simulink model "untitled"  (Simulink 7.5)
settings: Solver=ode45  StartTime=0.0  StopTime=100.0  RelTol=1e-3
settings Model: Creator=psoltysiak  LastModifiedBy=Soltys
settings DebuggingCC: StrictBusMsg=Warning

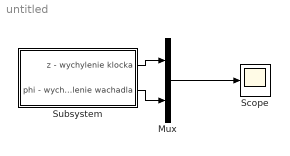
== system untitled ==
  Mux : Mux  Inputs=2
  Scope : Scope
  Subsystem : Subsystem  mask{mk=5, mw=1, l=1, g=9.81, c=1, k1=0, k2=0}
      mask prompts: mk "MASA KLOCKA"; mw "masa wahadla"; l "dlugosc wahadla"; g "przyspieszenie"; c "stala sprezyny"; k1 "wspolczynnik oporu klocka"; k2 "wspolczynnik ooru klocka"
  wires:
  Mux/1 -> Scope/1
  Subsystem/1(z - wychylenie klocka) -> Mux/1
  Subsystem/2(phi - wychylenie wachadla) -> Mux/2

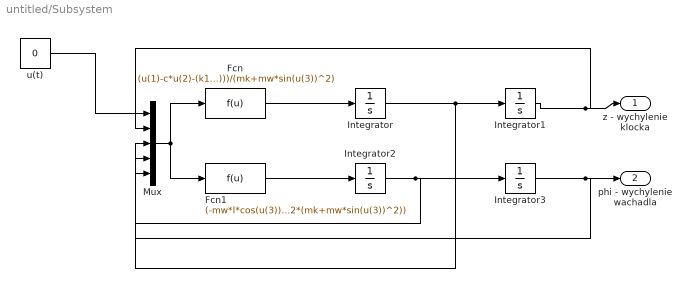
== system untitled/Subsystem ==
  Fcn : Fcn  Expr=(u(1)-c*u(2)-(k1+k2*sin(u(3))^2)*u(4)+mw*sin(u(3))*(l*u(5)^2+g*cos(u(3))))/(mk+mw*sin(u(3))^2)
  Fcn1 : Fcn  Expr=(-mw*l*cos(u(3))*(u(1))+mw*l*cos(u(3))*c*u(2)+l*cos(u(3))*(mw*k1-mk*k2)*u(4)-k2*l^2*(mk+mw*sin(u(3))^2)*u(5)-(mk+mw)*mw*g*l*sin(u(3))-mw^2*l^2*sin(u(3))*cos(u(3))*u(5)^2)/(mw*l^2*(mk+mw*sin(u(3))^2))
  Integrator : Integrator
  Integrator1 : Integrator  InitialCondition=0.01
  Integrator2 : Integrator
  Integrator3 : Integrator  InitialCondition=180*pi/180
  Mux : Mux  Inputs=5
  u(t) : Constant  Value=0  OutDataType=fixdt(1, 16)  OutScaling=2^0
  z - wychylenie klocka : Outport  OutDataType=fixdt(1, 16)  OutScaling=2^0
  phi - wychylenie wachadla : Outport  Port=2  OutDataType=fixdt(1, 16)  OutScaling=2^0
  wires:
  Fcn/1 -> Integrator/1
  Integrator/1 -> Integrator1/1, Mux/4
  Fcn1/1 -> Integrator2/1
  Integrator2/1 -> Integrator3/1, Mux/5
  Integrator1/1 -> z - wychylenie klocka/1, Mux/2
  Integrator3/1 -> phi - wychylenie wachadla/1, Mux/3
  Mux/1 -> Fcn/1, Fcn1/1
  u(t)/1 -> Mux/1
